simulink model "ECMO_Device_Project"  (R2020b)
settings: Solver=ode4  StartTime=0.0  StopTime=300  FixedStep=Tsamp  RelTol=1e-3
model workspace (MATLAB code in the model file):
  | %%%%%%%%%%%%%%%%%%%%%%%%%%%%%%%%%%%%%%%%%%%%%%%%%%%
  | %%%%%%%%%%%%% Term Project Parameters %%%%%%%%%%%%%
  | %%%%%%%%%%%%%%%%%%%%%%%%%%%%%%%%%%%%%%%%%%%%%%%%%%%
  | 
  | %% Physiological/Environmental Parameters
  | Tsamp = 1e-3;      % s
  | FIO2 = 50/100;  % (%) (Change this to 50% when ECMO is initiated)
  | FICO2 = 0.0/100;   % (%)
  | Patm = 760.0;      % mmHg
  | Pws = 47.0;        % mmHg
  | shunt = 36.5/100;  % (%)
  | 
  | %% Parameters of the Lung Mechanics
  | Clung = 0.062;     % l/cmH2O
  | Rtube = 3.76;      % cmH2O.s.l^-1
  | Rlung = 1.4013;    % cmH2O.s.l^-1
  | VL0 = 3.40;        % l
  | VReference = 0.2;  % l  (Change this to 0.2 l when ECMO is initiated)
  | 
  | %% Parameters of the Dead-Space
  | VD = 0.15;         % l
  | PdO2_IC = 60.0;    % mmHg
  | PdCO2_IC = 53.0;   % mmHg
  | 
  | %% Parameters of the Alveolar Gas Exchange
  | PAO2_IC = 57.0;    % mmHg
  | PACO2_IC = 55.0;   % mmHg
  | CaO2_IC = 0.184;   % ml/ml
  | CaCO2_IC = 0.565;  % ml/ml
  | Tau_TL = 10.0;     % s
  | kEff = 0.55;
  | 
  | %% Parameters of the Blood Dissociation Curves
  | CsatO2 = 0.2128;   % ml/ml
  | alpha1 = 0.03198;  % mmHg^-1
  | beta1 = 0.008275;  % mmHg^-1
  | K1 = 15.0;         % mmHg
  | h1 = 0.3836;
  | 
  | CsatCO2 = 1.9488;  % ml/ml
  | alpha2 = 0.05591;  % mmHg^-1
  | beta2 = 0.03255;   % mmHg^-1
  | K2 = 194.4;        % mmHg
  | h2 = 1.819;
  | 
  | %% Parameters of the Tissue Gas Exchange
  | VTO2 = 7700;       % ml
  | VTCO2 = 6000;      % ml
  | MRO2 = 3.80;       % ml/s
  | MRCO2 = 3.30;      % ml/s
  | CvO2_IC = 0.134;   % ml/ml
  | CvCO2_IC = 0.602;  % ml/ml
  | Tau_LT = 18.0;     % s
  | 
  | %% ECMO Pump Parameters
  | R = 10.0;     % ohm
  | L = 10.0;     % mH
  | kem = 0.192;  % V/(rd/s)
  | JL = 8e-4;    % kg.m^2
  | Ng = 0.5;
  | 
  | %% ECMO Oxygenator Parameters
  | VEO2 = 1.5;       % l
  | VECO2 = 1.5;      % l
  | PEO2_IC = 200.0;  % mmHg
  | PECO2_IC = 40.0;  % mmHg
  | 
  | FIEO2 = 100/100;   % (%)
  |  % (Change this to initiate ECMO)
libraries: fl_lib x19, nesl_utility x7, pid_lib x4
(part 1 of 2)
settings Model: OrderedModelArguments=off  Creator=kagan  LastModifiedBy=90535

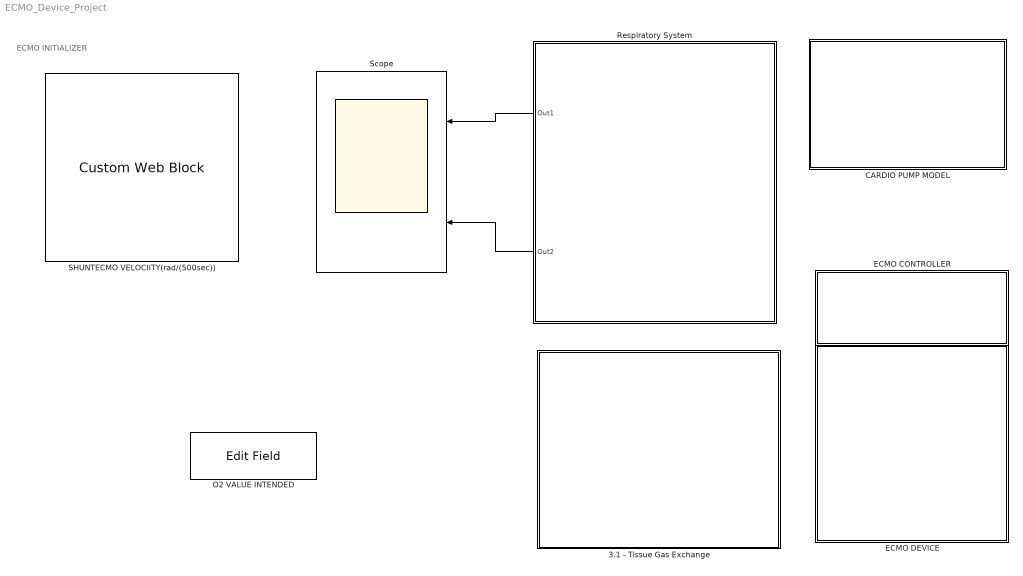
== system ECMO_Device_Project ==
  note: ECMO INITIALIZER
  3.1 - Tissue Gas Exchange : Subsystem
  CARDIO PUMP MODEL : Subsystem
  ECMO CONTROLLER : Subsystem
  ECMO DEVICE : Subsystem
  O2 VALUE INTENDED : EditField  LabelPosition=Hide  ShowInitialText=on  Alignment=Center
  Respiratory System : Subsystem
  SHUNTECMO VELOCIITY(rad/(500sec)) : CustomWebBlock  ShowInitialText=on  Configuration="{\"components\":[{\"name\":\"CircularScaleComponent\",\"settings\":{\"bounds\":{\"max\":1,\"min\":0,\"tickInterval\":\"auto\"},\"direction\":\"cw\",\"flipLimits\":0,\"innerRadius\":0.5069579852213397,\"internalTickHeightScaleFactor\":1,\"labelColor\":[250,245,200],\"labelFont\":{\"font\":\"Arial\",\"fontSize\":12},\"labelTransparency\":1,\"labelTrasparency\":1,\"minorTickHeightScaleFactor\":0.2,\"needleImage\":{\"size\":[200,50],\"src\":\"data:image\\/svg+xml;base64,PD94bWwgdmVyc2lvbj0iMS4wIiBlbmNvZGluZz0idXRmLTgiPz4KPCEtLSBHZW5lcmF0b3I6IEFkb2JlIElsbHVzdHJhdG9yIDE5LjIuMSwgU1ZHIEV4cG9ydCBQbHVnLUluIC4gU1ZHIFZlcnNpb246IDYuMDAgQnVpbGQgMCkgIC0tPgo8c3ZnIHZlcnNpb249IjEuMSIgeG1sbnM9Imh0dHA6Ly93d3cudzMub3JnLzIwMDAvc3ZnIiB4bWxuczp4bGluaz0iaHR0cDovL3d3dy53My5vcmcvMTk5OS94bGluayIgeD0iMHB4IiB5PSIwcHgiCgkgdmlld0JveD0iMCAwIDIwMCA1MCIgc3R5bGU9ImVuYWJsZS1iYWNrZ3JvdW5kOm5ldyAw ...(+9940 chars)\"},\"needleOffset\":[0.086575214380406,0],\"needleOrientation\":-45,\"needleRotation\":-180,\"needleSize\":{\"height\":0.09176649447596184,\"width\":0.3593006118373072},\"outerRadius\":0.6806022064516383,\"position\":[0.06486742424242424,0.05627705627705628,0.8917748917748918,0.8787878787878788],\"scaleAngle\":299.999999999988,\"scaleAngleOffset\":119.46147497096791,\"scaleColors\":[],\"scaleColorsSize\":0.2,\"scalePosition\":[0,0,1,1],\"showLabels\":1,\"showMinorTicks\":1,\"showSpanLine\":1,\"showTicks\":1,\"tickColor\":[250,245,200],\"tickTransparency\":1,\"valueBarColor\":[23,89,176],\"valueBarPosition\":[0,0,1,1],\"valueBarSize\":0.2,\"valueBarTransparency\":1}},{\"name\":\"BackgroundImageComponent\",\"settings\":{\"image\":{\"size\":[500,500],\"src\":\"data:image\\/svg+xml;base64,PD94bWwgdmVyc2lvbj0iMS4wIiBlbmNvZGluZz0iVVRGLTgiIHN0YW5kYWxvbmU9Im5vIj8+CjwhLS0gR2VuZXJhdG9yOiBBZG9iZSBJbGx1c3RyYXRvciAxOS4yLjEsIFNWRyBFeHBvcnQgUGx1Zy1JbiAuIFNWRyBWZXJzaW9uOiA2LjAwIEJ1aWxkIDApICAtLT4KCjxzdmcKICAgeG1sbnM6ZGM9Imh0dHA6Ly9wdXJsLm9yZy9kYy9lbGVtZW50cy8xLjEvIgogICB4bWxuczpjYz0iaHR0cDovL2NyZWF0aXZlY29tbW9ucy5vcmcvbnMjIgogICB4bWxuczpyZGY9Imh0dHA6Ly93d3cudzMub3JnLzE5OTkvMDIvMjItcmRmLXN5bnRh ...(+9660 chars)\",\"srcOrientation\":\"horizontal\"},\"position\":[0,0,1,1],\"scaleMode\":\"0\"}},{\"name\":\"ForegroundImageComponent\",\"settings\":{\"image\":{\"size\":[0,0],\"src\":\"default\",\"srcOrientation\":[]},\"isForeground\":1,\"position\":[0,0,1,1],\"scaleMode\":\"0\"}}],\"settings\":{\"BindingType\":\"signal\",\"aspectRatio\":1.0216110019646365,\"fixedAspectRatio\":\"on\",\"orientation\":\"horizontal\"},\"type\":\"CircularGauge\"}"
  Scope : Scope  NumInputPorts=2
  wires:
  Respiratory System/1(Out1) -> Scope/1
  Respiratory System/2(Out2) -> Scope/2

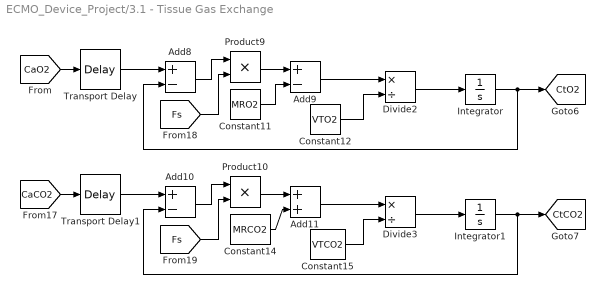
== system ECMO_Device_Project/3.1 - Tissue Gas Exchange ==
  Add10 : Sum  Inputs=+-
  Add11 : Sum
  Add8 : Sum  Inputs=+-
  Add9 : Sum  Inputs=+-
  Constant11 : Constant  Value=MRO2  SampleTime=Tsamp
  Constant12 : Constant  Value=VTO2  SampleTime=Tsamp
  Constant14 : Constant  Value=MRCO2  SampleTime=Tsamp
  Constant15 : Constant  Value=VTCO2  SampleTime=Tsamp
  Divide2 : Product  Inputs=*/
  Divide3 : Product  Inputs=*/
  Integrator : Integrator  InitialCondition=CvO2_IC
  Integrator1 : Integrator  InitialCondition=CvCO2_IC
  Product10 : Product
  Product9 : Product
  Transport Delay : TransportDelay  DelayTime=Tau_LT  InitialOutput=CaO2_IC
  Transport Delay1 : TransportDelay  DelayTime=Tau_LT  InitialOutput=CaCO2_IC
  tag scope: CtCO2=global, CtO2=global
  wires:
  [Fs] -> Product9/2
  Constant14/1 -> Add11/2
  [CaO2] -> Transport Delay/1
  Divide2/1 -> Integrator/1
  Integrator/1 -> Add8/2, [CtO2]
  Add8/1 -> Product9/1
  Add9/1 -> Divide2/1
  Divide3/1 -> Integrator1/1
  Constant12/1 -> Divide2/2
  Transport Delay/1 -> Add8/1
  Product9/1 -> Add9/1
  Constant11/1 -> Add9/2
  [CaCO2] -> Transport Delay1/1
  Integrator1/1 -> Add10/2, [CtCO2]
  Add11/1 -> Divide3/1
  Product10/1 -> Add11/1
  Transport Delay1/1 -> Add10/1
  Constant15/1 -> Divide3/2
  Add10/1 -> Product10/1
  [Fs] -> Product10/2

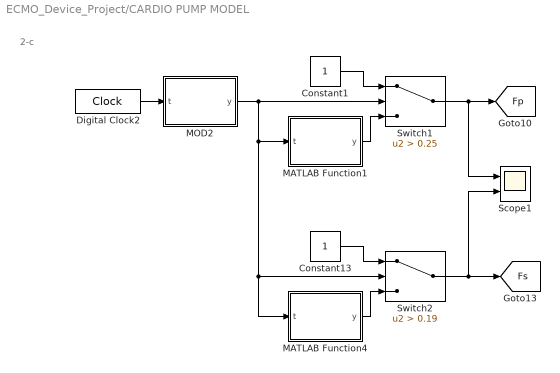
== system ECMO_Device_Project/CARDIO PUMP MODEL ==
  note: 2-c
  Constant1 : Constant
  Constant13 : Constant
  Digital Clock2 : DigitalClock  SampleTime=0.001
  MATLAB Function1 : MATLAB Function  TreatAsAtomicUnit=on
  MATLAB Function4 : MATLAB Function  TreatAsAtomicUnit=on
  MOD2 : MATLAB Function  TreatAsAtomicUnit=on
  Scope1 : Scope  NumInputPorts=2
  Switch1 : Switch  Criteria=u2 > Threshold  Threshold=0.25
  Switch2 : Switch  Criteria=u2 > Threshold  Threshold=0.19
  tag scope: Fp=global, Fs=global
  wires:
  Constant13/1 -> Switch2/1
  MOD2/1(y) -> MATLAB Function4/1(t), Switch2/2, MATLAB Function1/1(t), Switch1/2
  Switch1/1 -> [Fp], Scope1/1
  Switch2/1 -> Scope1/2, [Fs]
  Digital Clock2/1 -> MOD2/1(t)
  MATLAB Function4/1(y) -> Switch2/3
  Constant1/1 -> Switch1/1
  MATLAB Function1/1(y) -> Switch1/3

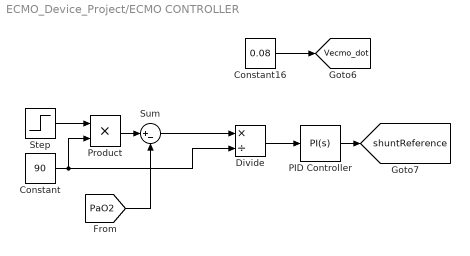
== system ECMO_Device_Project/ECMO CONTROLLER ==
  Constant : Constant  Value=90
  Constant16 : Constant  Value=0.08
  Divide : Product  Inputs=*/
  PID Controller : pid_lib/PID Controller  Controller=PI  Form=Parallel  TimeDomain=Continuous-time  UseExternalTs=off  SampleTime=-1  IntegratorMethod=Forward Euler  FilterMethod=Forward Euler  ControllerParametersSource=internal  P=10  I=4  D=600  UseFilter=on  N=100  TunerSelectOption=Transfer Function Based (PID Tuner App)  InitialConditionSource=internal  InitialConditionForIntegrator=0  InitialConditionForFilter=0  DifferentiatorICPrevScaledInput=0  ExternalReset=none  TrackingMode=off  Kt=1  LimitOutput=on  SatLimitsSource=internal  UpperSaturationLimit=1  LowerSaturationLimit=0  LinearizeAsGain=on  AntiWindupMode=none  Kb=1  POutMin=[]  POutMax=[]  IOutMin=[]  IOutMax=[]  DOutMin=[]  DOutMax=[]  NOutMin=[]  NOutMax=[]  SumOutMin=[]  SumOutMax=[]  SaturationOutMin=[]  SaturationOutMax=[]  PParamMin=[]  PParamMax=[]  IParamMin=[]  IParamMax=[]  DParamMin=[]  DParamMax=[]  NParamMin=[]  NParamMax=[]  KbParamMin=[]  KbParamMax=[]  KtParamMin=[]  KtParamMax=[]  KbOutMin=[]  KbOutMax=[]  KtOutMin=[]  KtOutMax=[]  IntegratorOutMin=[]  IntegratorOutMax=[]  FilterOutMin=[]  FilterOutMax=[]  SumI1OutMin=[]  SumI1OutMax=[]  SumI2OutMin=[]  SumI2OutMax=[]  SumI3OutMin=[]  SumI3OutMax=[]  SumI4OutMin=[]  SumI4OutMax=[]  SumDOutMin=[]  SumDOutMax=[]  DifferentiatorOutMin=[]  DifferentiatorOutMax=[]  FilterDiffOutCoefMin=[]  FilterDiffOutCoefMax=[]  ReciprocalOutMin=[]  ReciprocalOutMax=[]  SumDenOutMin=[]  SumDenOutMax=[]  SumNumOutMin=[]  SumNumOutMax=[]  DivideOutMin=[]  DivideOutMax=[]  UdiffTsProdOutMin=[]  UdiffTsProdOutMax=[]  NTsProdOutMin=[]  NTsProdOutMax=[]  UintegralTsProdOutMin=[]  UintegralTsProdOutMax=[]  UngainTsProdOutMin=[]  UngainTsProdOutMax=[]  IntegratorContinuousStateAttributes=''  IntegratorStateMustResolveToSignalObject=off  IntegratorRTWStateStorageClass=Auto  FilterContinuousStateAttributes=''  FilterStateMustResolveToSignalObject=off  FilterRTWStateStorageClass=Auto  ParallelPVariant=InternalParameters  IdealPVariant=Disabled  IVariant=InternalParameters  DVariant=Disabled  IntegratorVariant=Continuous  SatVariant=Enabled  AWVariant=Passthrough  PCopyVariant=Disabled  TRVariant=Disabled  FdbkBlocksVariant=Forward  IdealPFdbkVariant=Disabled  SatFdbkVariant=Disabled  DerivativeFilterVariant=Disabled  NVariant=Disabled  NCopyVariant=Disabled_SignalSpec  FilterICVariant=Disabled  IntegratorICVariant=InternalICs  ExternalResetVariant=Disabled  TRSumVariant=Passthrough  SumFdbkVariant=Disabled  SumVariant=Sum_PI  TsampFilterVariant=InternalTs  TsampNgainVariant=Passthrough  TsampIntegralVariant=Passthrough  ExternalSaturationOutDataTypeStr=Inherit: Same as second input
  Product : Product
  Step : Step  Time=0  SampleTime=0
  Sum : Sum  Inputs=|+-
  tag scope: Vecmo_dot=global, shuntReference=global
  wires:
  Product/1 -> Sum/1
  [PaO2] -> Sum/2
  PID Controller/1 -> [shuntReference]
  Constant16/1 -> [Vecmo_dot]
  Sum/1 -> Divide/1
  Divide/1 -> PID Controller/1
  Constant/1 -> Divide/2, Product/2
  Step/1 -> Product/1

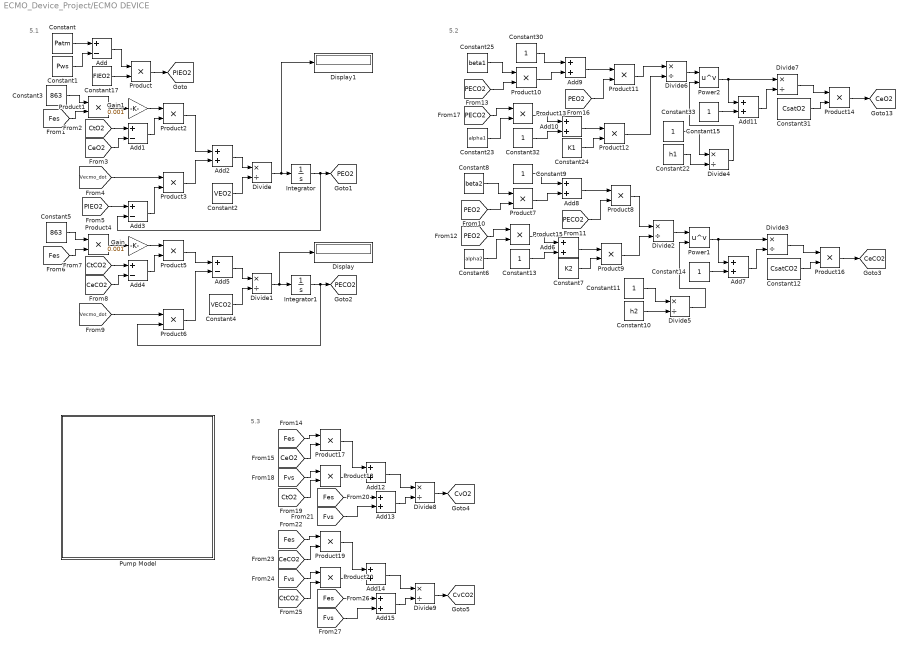
== system ECMO_Device_Project/ECMO DEVICE ==
  note: 5.3
  note: 5.1
  note: 5.2
  Add{,1,3..5} (5 alike) : Sum  Inputs=+-
  Add{2,6..15} (11 alike) : Sum
  Constant : Constant  Value=Patm
  Constant1 : Constant  Value=Pws
  Constant10 : Constant  Value=h2  SampleTime=Tsamp
  Constant{9,11,13..15,30,32..33} (8 alike) : Constant  SampleTime=Tsamp
  Constant12 : Constant  Value=CsatCO2  SampleTime=Tsamp
  Constant17 : Constant  Value=FIEO2
  Constant2 : Constant  Value=VEO2
  Constant22 : Constant  Value=h1  SampleTime=Tsamp
  Constant23 : Constant  Value=alpha1  SampleTime=Tsamp
  Constant24 : Constant  Value=K1  SampleTime=Tsamp
  Constant25 : Constant  Value=beta1  SampleTime=Tsamp
  Constant3 : Constant  Value=863
  Constant31 : Constant  Value=CsatO2  SampleTime=Tsamp
  Constant4 : Constant  Value=VECO2
  Constant5 : Constant  Value=863
  Constant6 : Constant  Value=alpha2  SampleTime=Tsamp
  Constant7 : Constant  Value=K2  SampleTime=Tsamp
  Constant8 : Constant  Value=beta2  SampleTime=Tsamp
  Display : Display
  Display1 : Display
  Divide{,1..9} (10 alike) : Product  Inputs=*/
  Gain : Gain  Gain=0.001
  Gain1 : Gain  Gain=0.001
  Integrator : Integrator  InitialCondition=PEO2_IC
  Integrator1 : Integrator  InitialCondition=PECO2_IC
  Power1 : Math  Operator=pow  SaturateOnIntegerOverflow=on
  Power2 : Math  Operator=pow  SaturateOnIntegerOverflow=on
  Product{,1..20} (21 alike) : Product
  "Pump Model " : Subsystem
  tag scope: CeCO2=global, CeO2=global, CvCO2=global, CvO2=global, PECO2=global, PEO2=global, PIEO2=global
  wires:
  [PECO2] -> Product8/2
  Constant2/1 -> Divide/2
  Product11/1 -> Divide6/1
  Divide4/1 -> Power2/2
  Constant15/1 -> Divide4/1
  Product7/1 -> Add8/2
  [Fes] -> Add13/1
  Add12/1 -> Divide8/1
  Gain/1 -> Product5/1
  Constant13/1 -> Add6/2
  Product20/1 -> Add14/2
  [Fvs] -> Add15/2
  [Fes] -> Product19/1
  Constant3/1 -> Product1/1
  [Fes] -> Product17/1
  [PECO2] -> Product10/2
  Power1/1 -> Add7/1, Divide3/1
  Add2/1 -> Divide/1
  Constant10/1 -> Divide5/2
  Add13/1 -> Divide8/2
  [CtO2] -> Product18/2
  Divide6/1 -> Power2/1
  Add3/1 -> Product3/2
  [PEO2] -> Product11/2
  Add10/1 -> Product12/1
  Divide1/1 -> Display/1, Integrator1/1
  [Fes] -> Product1/2
  Constant24/1 -> Product12/2
  Integrator1/1 -> Product6/2, [PECO2]
  Constant1/1 -> Add/2
  Constant6/1 -> Product15/2
  Integrator/1 -> Add3/2, [PEO2]
  Add11/1 -> Divide7/2
  Product8/1 -> Divide2/1
  Product17/1 -> Add12/1
  [Vecmo_dot] -> Product3/1
  [CtCO2] -> Add4/1
  Constant7/1 -> Product9/2
  Product18/1 -> Add12/2
  Product10/1 -> Add9/2
  Product14/1 -> [CeO2]
  Add4/1 -> Product5/2
  [PIEO2] -> Add3/1
  Product6/1 -> Add5/2
  Constant14/1 -> Add7/2
  Divide5/1 -> Power1/2
  Gain1/1 -> Product2/1
  Add9/1 -> Product11/1
  Product5/1 -> Add5/1
  Constant33/1 -> Add11/2
  Add15/1 -> Divide9/2
  Add8/1 -> Product8/1
  Constant11/1 -> Divide5/1
  [PEO2] -> Product15/1
  Constant5/1 -> Product4/1
  Constant17/1 -> Product/2
  Constant31/1 -> Product14/2
  Divide3/1 -> Product16/1
  Divide/1 -> Display1/1, Integrator/1
  Add1/1 -> Product2/2
  Add7/1 -> Divide3/2
  Add/1 -> Product/1
  Constant/1 -> Add/1
  Power2/1 -> Add11/1, Divide7/1
  Add5/1 -> Divide1/1
  Constant12/1 -> Product16/2
  Product9/1 -> Divide2/2
  Product16/1 -> [CeCO2]
  Constant32/1 -> Add10/2
  Product12/1 -> Divide6/2
  Product3/1 -> Add2/2
  Divide2/1 -> Power1/1
  [Fvs] -> Product18/1
  [CeCO2] -> Product19/2
  [Fes] -> Product4/2
  Add14/1 -> Divide9/1
  Divide8/1 -> [CvO2]
  Constant9/1 -> Add8/1
  [CtO2] -> Add1/1
  [Fvs] -> Add13/2
  Divide7/1 -> Product14/1
  Constant4/1 -> Divide1/2
  Divide9/1 -> [CvCO2]
  Constant8/1 -> Product7/1
  Add6/1 -> Product9/1
  Product1/1 -> Gain1/1
  Constant30/1 -> Add9/1
  Product2/1 -> Add2/1
  Product15/1 -> Add6/1
  Product/1 -> [PIEO2]
  Constant25/1 -> Product10/1
  [PECO2] -> Product13/1
  Constant23/1 -> Product13/2
  [CeO2] -> Product17/2
  Product4/1 -> Gain/1
  Product13/1 -> Add10/1
  [Fvs] -> Product20/1
  Constant22/1 -> Divide4/2
  [CeO2] -> Add1/2
  [PEO2] -> Product7/2
  [Vecmo_dot] -> Product6/1
  [CeCO2] -> Add4/2
  [CtCO2] -> Product20/2
  [Fes] -> Add15/1
  Product19/1 -> Add14/1

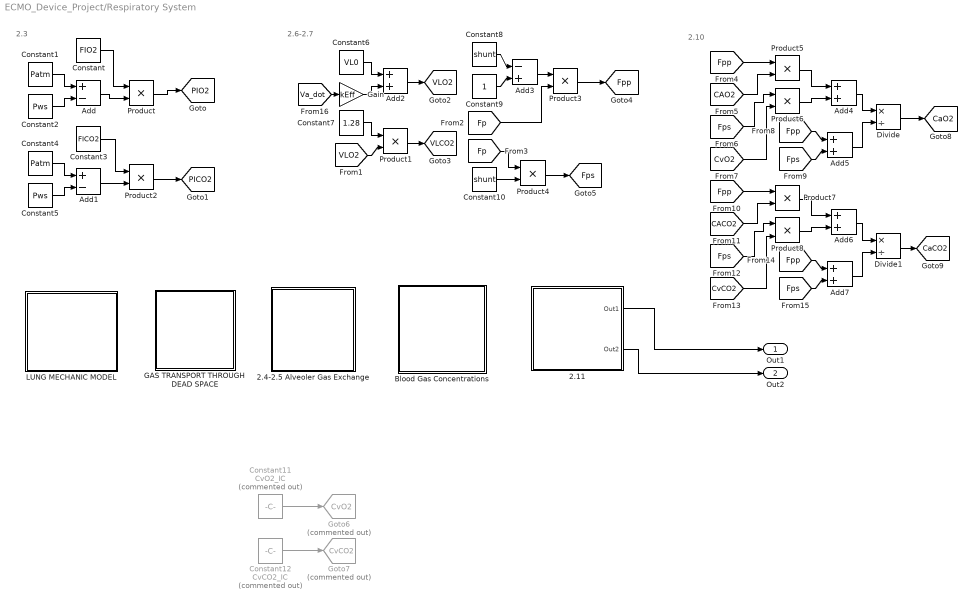
== system ECMO_Device_Project/Respiratory System ==
  note: 2.10
  note: 2.6-2.7
  note: 2.3
  "2.11 " : Subsystem
  2.4-2.5 Alveoler Gas Exchange : Subsystem
  Add : Sum  Inputs=+-
  Add1 : Sum  Inputs=+-
  Add{2,4..7} (5 alike) : Sum
  Add3 : Sum  Inputs=-+
  "Blood Gas Concentrations " : Subsystem
  Constant : Constant  Value=FIO2  SampleTime=Tsamp
  Constant1 : Constant  Value=Patm  SampleTime=Tsamp
  Constant10 : Constant  Value=shunt  SampleTime=Tsamp
  Constant11 : Constant  Commented=on  Value=CvO2_IC  SampleTime=Tsamp
  Constant12 : Constant  Commented=on  Value=CvCO2_IC  SampleTime=Tsamp
  Constant2 : Constant  Value=Pws  SampleTime=Tsamp
  Constant3 : Constant  Value=FICO2  SampleTime=Tsamp
  Constant4 : Constant  Value=Patm  SampleTime=Tsamp
  Constant5 : Constant  Value=Pws  SampleTime=Tsamp
  Constant6 : Constant  Value=VL0  SampleTime=Tsamp
  Constant7 : Constant  Value=1.28  SampleTime=Tsamp
  Constant8 : Constant  Value=shunt  SampleTime=Tsamp
  Constant9 : Constant  SampleTime=Tsamp
  Divide : Product  Inputs=*/
  Divide1 : Product  Inputs=*/
  GAS TRANSPORT THROUGH DEAD SPACE : Subsystem
  Gain : Gain  Gain=kEff
  Goto6 : Goto  Commented=on  GotoTag=CvO2  TagVisibility=global
  Goto7 : Goto  Commented=on  GotoTag=CvCO2  TagVisibility=global
  LUNG MECHANIC MODEL : Subsystem
  Product{,1..8} (9 alike) : Product
  Out1 : Outport
  Out2 : Outport  Port=2
  tag scope: CaCO2=global, CaO2=global, Fpp=global, Fps=global, PICO2=global, PIO2=global, VLCO2=global, VLO2=global
  wires:
  Constant9/1 -> Add3/2
  Add5/1 -> Divide/2
  Constant2/1 -> Add/2
  Constant10/1 -> Product4/2
  Constant8/1 -> Add3/1
  Add4/1 -> Divide/1
  [Fp] -> Product3/2
  Add2/1 -> [VLO2]
  [CvO2] -> Product6/2
  Constant5/1 -> Add1/2
  Constant7/1 -> Product1/1
  [VLO2] -> Product1/2
  Constant3/1 -> Product2/1
  [Fp] -> Product4/1
  Add3/1 -> Product3/1
  Constant1/1 -> Add/1
  Product5/1 -> Add4/1
  Product8/1 -> Add6/2
  Constant4/1 -> Add1/1
  Product3/1 -> [Fpp]
  Gain/1 -> Add2/2
  [Fps] -> Add7/2
  Product1/1 -> [VLCO2]
  [Fpp] -> Add7/1
  Product2/1 -> [PICO2]
  Add/1 -> Product/2
  Add1/1 -> Product2/2
  Constant6/1 -> Add2/1
  Add6/1 -> Divide1/1
  [CvCO2] -> Product8/2
  [CACO2] -> Product7/2
  Product6/1 -> Add4/2
  [CAO2] -> Product5/2
  Product4/1 -> [Fps]
  [Fpp] -> Add5/1
  Constant/1 -> Product/1
  Product7/1 -> Add6/1
  Divide1/1 -> [CaCO2]
  Product/1 -> [PIO2]
  [Va_dot] -> Gain/1
  [Fps] -> Product8/1
  [Fpp] -> Product5/1
  [Fps] -> Add5/2
  Add7/1 -> Divide1/2
  [Fps] -> Product6/1
  [Fpp] -> Product7/1
  Divide/1 -> [CaO2]
  Constant11/1 -> Goto6/1
  Constant12/1 -> Goto7/1
  "2.11 "/1(Out1) -> Out1/1
  "2.11 "/2(Out2) -> Out2/1

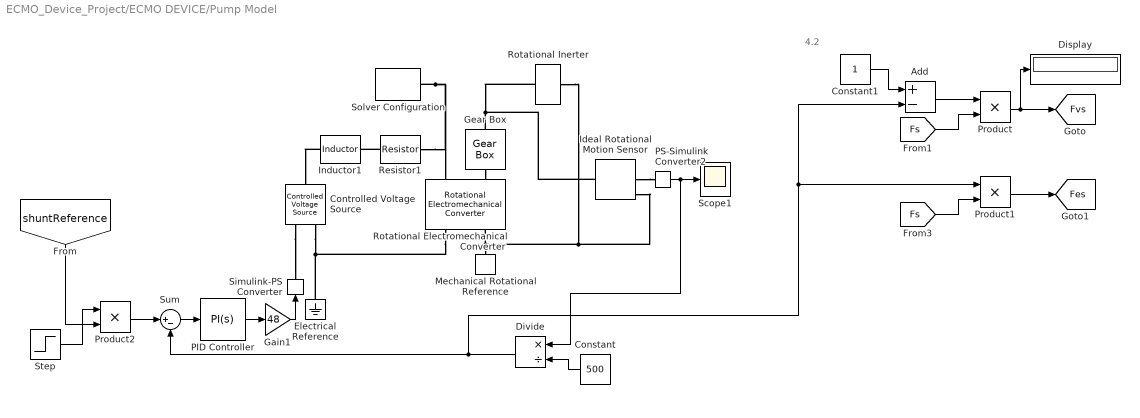
== system ECMO_Device_Project/ECMO DEVICE/Pump Model  ==
  note: 4.2
  Add : Sum  Inputs=+-
  Constant : Constant  Value=500
  Constant1 : Constant
  Controlled Voltage Source : fl_lib/Electrical/Electrical Sources/Controlled Voltage Source
  Display : Display
  Divide : Product  Inputs=*/
  Electrical Reference : fl_lib/Electrical/Electrical Elements/Electrical Reference
  Gain1 : Gain  Gain=48
  Gear Box : fl_lib/Mechanical/Mechanisms/Gear Box  ratio=Ng  t_in_specify=off  t_in_priority=None  t_in=0 N*m  t_in_nominal_specify=off  t_in_nominal_unit=N*m  t_in_nominal_value=1  t_out_specify=off  t_out_priority=None  t_out=0 N*m  t_out_nominal_specify=off  t_out_nominal_unit=N*m  t_out_nominal_value=1
  Ideal Rotational Motion Sensor : fl_lib/Mechanical/Mechanical Sensors/Ideal Rotational Motion Sensor  wrap_angle=simscape.enum.onoff.off  offset=0 rad
  Inductor1 : fl_lib/Electrical/Electrical Elements/Inductor  l=L mH  r=0 Ohm  g=1e-9 1/Ohm  i_specify=off  i_priority=None  i=0 A  i_nominal_specify=off  i_nominal_unit=A  i_nominal_value=1  v_specify=off  v_priority=None  v=0 V  v_nominal_specify=off  v_nominal_unit=V  v_nominal_value=1  i_L_specify=off  i_L_priority=High  i_L=0 A  i_L_nominal_specify=off  i_L_nominal_unit=A  i_L_nominal_value=1
  Mechanical Rotational Reference : fl_lib/Mechanical/Rotational Elements/Mechanical Rotational Reference
  PID Controller : pid_lib/PID Controller  Controller=PI  Form=Parallel  TimeDomain=Continuous-time  UseExternalTs=off  SampleTime=-1  IntegratorMethod=Forward Euler  FilterMethod=Forward Euler  ControllerParametersSource=internal  P=300  I=48.35  D=0  UseFilter=on  N=100  TunerSelectOption=Transfer Function Based (PID Tuner App)  InitialConditionSource=internal  InitialConditionForIntegrator=0  InitialConditionForFilter=0  DifferentiatorICPrevScaledInput=0  ExternalReset=none  TrackingMode=off  Kt=1  LimitOutput=on  SatLimitsSource=internal  UpperSaturationLimit=1  LowerSaturationLimit=0  LinearizeAsGain=on  AntiWindupMode=none  Kb=1  POutMin=[]  POutMax=[]  IOutMin=[]  IOutMax=[]  DOutMin=[]  DOutMax=[]  NOutMin=[]  NOutMax=[]  SumOutMin=[]  SumOutMax=[]  SaturationOutMin=[]  SaturationOutMax=[]  PParamMin=[]  PParamMax=[]  IParamMin=[]  IParamMax=[]  DParamMin=[]  DParamMax=[]  NParamMin=[]  NParamMax=[]  KbParamMin=[]  KbParamMax=[]  KtParamMin=[]  KtParamMax=[]  KbOutMin=[]  KbOutMax=[]  KtOutMin=[]  KtOutMax=[]  IntegratorOutMin=[]  IntegratorOutMax=[]  FilterOutMin=[]  FilterOutMax=[]  SumI1OutMin=[]  SumI1OutMax=[]  SumI2OutMin=[]  SumI2OutMax=[]  SumI3OutMin=[]  SumI3OutMax=[]  SumI4OutMin=[]  SumI4OutMax=[]  SumDOutMin=[]  SumDOutMax=[]  DifferentiatorOutMin=[]  DifferentiatorOutMax=[]  FilterDiffOutCoefMin=[]  FilterDiffOutCoefMax=[]  ReciprocalOutMin=[]  ReciprocalOutMax=[]  SumDenOutMin=[]  SumDenOutMax=[]  SumNumOutMin=[]  SumNumOutMax=[]  DivideOutMin=[]  DivideOutMax=[]  UdiffTsProdOutMin=[]  UdiffTsProdOutMax=[]  NTsProdOutMin=[]  NTsProdOutMax=[]  UintegralTsProdOutMin=[]  UintegralTsProdOutMax=[]  UngainTsProdOutMin=[]  UngainTsProdOutMax=[]  IntegratorContinuousStateAttributes=''  IntegratorStateMustResolveToSignalObject=off  IntegratorRTWStateStorageClass=Auto  FilterContinuousStateAttributes=''  FilterStateMustResolveToSignalObject=off  FilterRTWStateStorageClass=Auto  ParallelPVariant=InternalParameters  IdealPVariant=Disabled  IVariant=InternalParameters  DVariant=Disabled  IntegratorVariant=Continuous  SatVariant=Enabled  AWVariant=Passthrough  PCopyVariant=Disabled  TRVariant=Disabled  FdbkBlocksVariant=Forward  IdealPFdbkVariant=Disabled  SatFdbkVariant=Disabled  DerivativeFilterVariant=Disabled  NVariant=Disabled  NCopyVariant=Disabled_SignalSpec  FilterICVariant=Disabled  IntegratorICVariant=InternalICs  ExternalResetVariant=Disabled  TRSumVariant=Passthrough  SumFdbkVariant=Disabled  SumVariant=Sum_PI  TsampFilterVariant=InternalTs  TsampNgainVariant=Passthrough  TsampIntegralVariant=Passthrough  ExternalSaturationOutDataTypeStr=Inherit: Same as second input
  PS-Simulink Converter2 : nesl_utility/PS-Simulink Converter  PhysicalDomain=network_engine_domain  SubClassName=ps_output  LeftPortType=input  RightPortType=output  PseudoPeriodic=off  Frequencies=[]  Unit=inherit  AffineConversion=off
  Product : Product
  Product1 : Product
  Product2 : Product
  Resistor1 : fl_lib/Electrical/Electrical Elements/Resistor  R=R Ohm  i_specify=off  i_priority=None  i=0 A  i_nominal_specify=off  i_nominal_unit=A  i_nominal_value=1  v_specify=off  v_priority=None  v=0 V  v_nominal_specify=off  v_nominal_unit=V  v_nominal_value=1
  Rotational Electromechanical Converter : fl_lib/Electrical/Electrical Elements/Rotational Electromechanical Converter  K=kem V/(rad/s)  i_specify=off  i_priority=None  i=0 A  i_nominal_specify=off  i_nominal_unit=A  i_nominal_value=1  v_specify=off  v_priority=None  v=0 V  v_nominal_specify=off  v_nominal_unit=V  v_nominal_value=1  t_specify=off  t_priority=None  t=0 N*m  t_nominal_specify=off  t_nominal_unit=N*m  t_nominal_value=1  w_specify=off  w_priority=None  w=0 rad/s  w_nominal_specify=off  w_nominal_unit=rad/s  w_nominal_value=1
  Rotational Inerter : fl_lib/Mechanical/Rotational Elements/Rotational Inerter  B=JL kg*m^2  w_specify=off  w_priority=High  w=0 rad/s  w_nominal_specify=off  w_nominal_unit=rad/s  w_nominal_value=1  t_specify=off  t_priority=None  t=0 N*m  t_nominal_specify=off  t_nominal_unit=N*m  t_nominal_value=1
      settings: SourceProductBaseCode=SS  InternalSimscapePortConfiguration="{\"Bottom\":[],\"Left\":[{\"id\":\"R\",\"label\":\"R\",\"type\":\"foundation.mechanical.rotational.rotational\"}],\"Right\":[{\"id\":\"C\",\"label\":\"C\",\"type\":\"foundation.mechanical.rotational.rotational\"}],\"Top\":[]}"
  Scope1 : Scope
  Simulink-PS Converter : nesl_utility/Simulink-PS Converter  PhysicalDomain=network_engine_domain  SubClassName=ps_input  LeftPortType=input  RightPortType=output  PseudoPeriodic=off  Frequencies=[]  NoiseDistribution=none  NoiseParameters=[]  Unit=1  AffineConversion=off  FilteringAndDerivatives=provide  SimscapeFilterOrder=1  InputFilterTimeConstant=0.001  UdotUserProvided=0
  Solver Configuration : nesl_utility/Solver Configuration  PhysicalDomain=network_engine_domain  SubClassName=solver  LeftPortType=input  RightPortType=generic  Tones=[]  Harmonics=[]  SimulateNoise=off  Profile=off  UseLocalSampling=off  EnableSwitchedLinearOptims=on  FrequencyDomain=off  UseCCode=off  RelTol=0.001  AbsTol=1e-06  MinStep=1e-09  ToWorkspace=off  RevertToSquareIcSolve=off  NumHomotopyIterations=100  PhasorMode=off  PhasorModeNumHarmonics=1  DoDC=off  ResidualTolerance=1e-09  UseLocalSolver=off  LocalSolverChoice=NE_BACKWARD_EULER_ADVANCER  LocalSolverSampleTime=0.001  DoFixedCost=off  MaxNonlinIter=3  MaxModeIter=2  ComputeImpulses=off  ImpulseIterations=2  LinearAlgebra=auto  EquationFormulation=NE_TIME_EF  DelaysMemoryBudget=1024  AutomaticFiltering=on  FilteringTimeConstant=0.001  PartitionStorageMethod=AS_NEEDED  PartitionMemoryBudget=1024  PartitionMethod=ROBUST
  Step : Step  Time=0  SampleTime=0
  Sum : Sum  Inputs=|+-
  tag scope: Fes=global, Fvs=global
  wires:
  Sum/1 -> PID Controller/1
  Gain1/1 -> Simulink-PS Converter/1
  Constant/1 -> Divide/2
  PS-Simulink Converter2/1 -> Scope1/1, Divide/1
  Product2/1 -> Sum/1
  Step/1 -> Product2/1
  Divide/1 -> Product1/1, Add/2, Sum/2
  Constant1/1 -> Add/1
  Add/1 -> Product/1
  [Fs] -> Product/2
  Product/1 -> Display/1, [Fvs]
  PID Controller/1 -> Gain1/1
  [Fs] -> Product1/2
  Product1/1 -> [Fes]
  [shuntReference] -> Product2/2
  connections:
  Ideal Rotational Motion Sensor/RConn1 -- Mechanical Rotational Reference/LConn1 -- Rotational Electromechanical Converter/RConn2 -- Rotational Inerter/RConn1
  Controlled Voltage Source/RConn2 -- Rotational Electromechanical Converter/RConn1 -- Electrical Reference/LConn1
  Gear Box/LConn1 -- Rotational Electromechanical Converter/LConn2
  Gear Box/RConn1 -- Rotational Inerter/LConn1 -- Ideal Rotational Motion Sensor/LConn1
  Solver Configuration/RConn1 -- Resistor1/RConn1 -- Rotational Electromechanical Converter/LConn1
  Ideal Rotational Motion Sensor/RConn2 -- PS-Simulink Converter2/LConn1
  Inductor1/LConn1 -- Controlled Voltage Source/LConn1
  Controlled Voltage Source/RConn1 -- Simulink-PS Converter/RConn1
  Resistor1/LConn1 -- Inductor1/RConn1

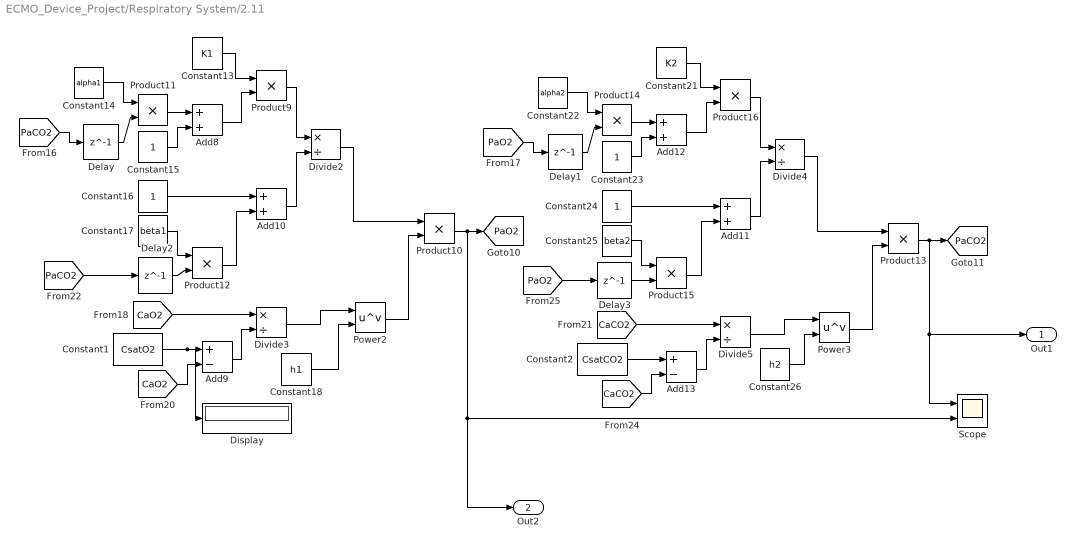
== system ECMO_Device_Project/Respiratory System/2.11  ==
  Add{8,10..12} (4 alike) : Sum
  Add13 : Sum  Inputs=+-
  Add9 : Sum  Inputs=+-
  Constant1 : Constant  Value=CsatO2  SampleTime=Tsamp
  Constant13 : Constant  Value=K1  SampleTime=Tsamp
  Constant14 : Constant  Value=alpha1  SampleTime=Tsamp
  Constant{15..16,23..24} (4 alike) : Constant  SampleTime=Tsamp
  Constant17 : Constant  Value=beta1  SampleTime=Tsamp
  Constant18 : Constant  Value=h1  SampleTime=Tsamp
  Constant2 : Constant  Value=CsatCO2  SampleTime=Tsamp
  Constant21 : Constant  Value=K2  SampleTime=Tsamp
  Constant22 : Constant  Value=alpha2  SampleTime=Tsamp
  Constant25 : Constant  Value=beta2  SampleTime=Tsamp
  Constant26 : Constant  Value=h2  SampleTime=Tsamp
  Delay : Delay  DelayLength=1  SampleTime=Tsamp
  Delay1 : Delay  DelayLength=1  InitialCondition=0  SampleTime=Tsamp
  Delay2 : Delay  DelayLength=1  InitialCondition=0  SampleTime=Tsamp
  Delay3 : Delay  DelayLength=1  InitialCondition=0  SampleTime=Tsamp
  Display : Display
  Divide{2..5} (4 alike) : Product  Inputs=*/
  Power2 : Math  Operator=pow  SaturateOnIntegerOverflow=on
  Power3 : Math  Operator=pow  SaturateOnIntegerOverflow=on
  Product{9..16} (8 alike) : Product
  Scope : Scope  NumInputPorts=2
  Out1 : Outport
  Out2 : Outport  Port=2
  tag scope: PaCO2=global, PaO2=global
  wires:
  Constant2/1 -> Add13/1
  Constant22/1 -> Product14/1
  [CaO2] -> Divide3/1
  Divide4/1 -> Product13/1
  Constant21/1 -> Product16/1
  Constant15/1 -> Add8/2
  Add12/1 -> Product16/2
  Add10/1 -> Divide2/2
  Product13/1 -> Out1/1, Scope/1, [PaCO2]
  Constant1/1 -> Display/1, Add9/1
  Add13/1 -> Divide5/2
  Product15/1 -> Add11/2
  Constant25/1 -> Product15/1
  [PaCO2] -> Delay/1
  Constant24/1 -> Add11/1
  Delay/1 -> Product11/2
  Delay1/1 -> Product14/2
  Product11/1 -> Add8/1
  [PaO2] -> Delay1/1
  Product10/1 -> Out2/1, Scope/2, [PaO2]
  [CaCO2] -> Add13/2
  Product12/1 -> Add10/2
  Product16/1 -> Divide4/1
  Constant14/1 -> Product11/1
  Power3/1 -> Product13/2
  Constant23/1 -> Add12/2
  [CaCO2] -> Divide5/1
  Add11/1 -> Divide4/2
  Product14/1 -> Add12/1
  Constant17/1 -> Product12/1
  Constant16/1 -> Add10/1
  Constant13/1 -> Product9/1
  Product9/1 -> Divide2/1
  Power2/1 -> Product10/2
  Add8/1 -> Product9/2
  [CaO2] -> Add9/2
  Divide2/1 -> Product10/1
  Add9/1 -> Divide3/2
  [PaCO2] -> Delay2/1
  Delay2/1 -> Product12/2
  Divide3/1 -> Power2/1
  Constant18/1 -> Power2/2
  Divide5/1 -> Power3/1
  Constant26/1 -> Power3/2
  [PaO2] -> Delay3/1
  Delay3/1 -> Product15/2

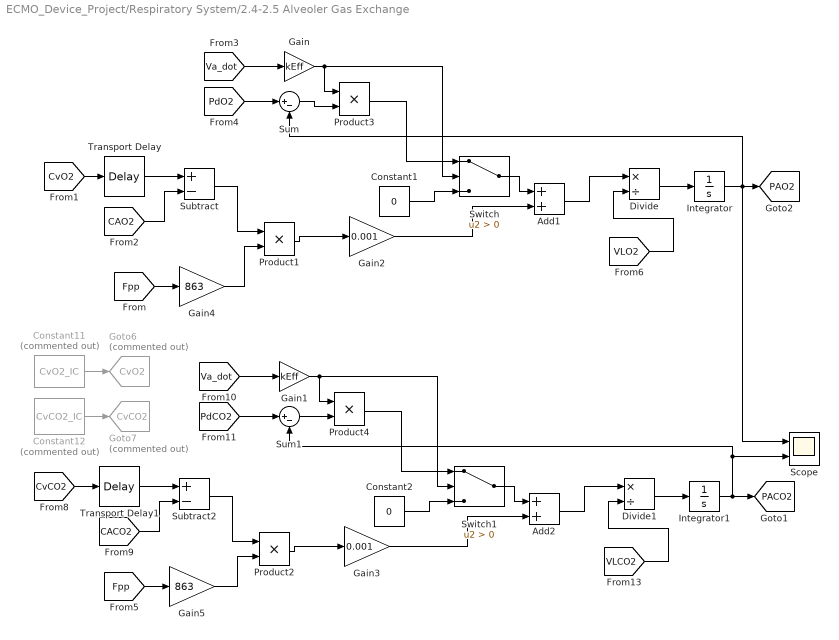
== system ECMO_Device_Project/Respiratory System/2.4-2.5 Alveoler Gas Exchange ==
  Add1 : Sum
  Add2 : Sum
  Constant1 : Constant  Value=0  SampleTime=Tsamp
  Constant11 : Constant  Commented=on  Value=CvO2_IC  SampleTime=Tsamp
  Constant12 : Constant  Commented=on  Value=CvCO2_IC  SampleTime=Tsamp
  Constant2 : Constant  Value=0  SampleTime=Tsamp
  Divide : Product  Inputs=*/
  Divide1 : Product  Inputs=*/
  Gain : Gain  Gain=kEff
  Gain1 : Gain  Gain=kEff
  Gain2 : Gain  Gain=0.001
  Gain3 : Gain  Gain=0.001
  Gain4 : Gain  Gain=863
  Gain5 : Gain  Gain=863
  Goto6 : Goto  Commented=on  GotoTag=CvO2  TagVisibility=global
  Goto7 : Goto  Commented=on  GotoTag=CvCO2  TagVisibility=global
  Integrator : Integrator  InitialCondition=PAO2_IC
  Integrator1 : Integrator  InitialCondition=PACO2_IC
  Product{1..4} (4 alike) : Product
  Scope : Scope  NumInputPorts=2
  Subtract : Sum  Inputs=+-
  Subtract2 : Sum  Inputs=+-
  Sum : Sum  Inputs=|+-
  Sum1 : Sum  Inputs=|+-
  Switch : Switch  Criteria=u2 > Threshold
  Switch1 : Switch  Criteria=u2 > Threshold
  Transport Delay : TransportDelay  DelayTime=Tau_TL  InitialOutput=CvO2_IC  BufferSize=10240  FixedBuffer=on
  Transport Delay1 : TransportDelay  DelayTime=Tau_TL  InitialOutput=CvCO2_IC  BufferSize=10240  FixedBuffer=on
  tag scope: PACO2=global, PAO2=global
  wires:
  Product3/1 -> Switch/1
  Subtract/1 -> Product1/1
  [CAO2] -> Subtract/2
  [Va_dot] -> Gain/1
  Gain/1 -> Product3/1, Switch/2
  Transport Delay/1 -> Subtract/1
  [CvO2] -> Transport Delay/1
  Divide/1 -> Integrator/1
  [PdO2] -> Sum/1
  Integrator/1 -> Sum/2, Scope/1, [PAO2]
  Sum/1 -> Product3/2
  [VLO2] -> Divide/2
  Product1/1 -> Gain2/1
  Constant1/1 -> Switch/3
  Switch/1 -> Add1/1
  Gain2/1 -> Add1/2
  Add1/1 -> Divide/1
  [PdCO2] -> Sum1/1
  [CvCO2] -> Transport Delay1/1
  Subtract2/1 -> Product2/1
  [CACO2] -> Subtract2/2
  Divide1/1 -> Integrator1/1
  Switch1/1 -> Add2/1
  Integrator1/1 -> Sum1/2, Scope/2, [PACO2]
  Transport Delay1/1 -> Subtract2/1
  Sum1/1 -> Product4/2
  Product4/1 -> Switch1/1
  Constant2/1 -> Switch1/3
  [VLCO2] -> Divide1/2
  Product2/1 -> Gain3/1
  Add2/1 -> Divide1/1
  [Va_dot] -> Gain1/1
  Gain3/1 -> Add2/2
  Gain1/1 -> Product4/1, Switch1/2
  [Fpp] -> Gain4/1
  Gain4/1 -> Product1/2
  Gain5/1 -> Product2/2
  [Fpp] -> Gain5/1
  Constant12/1 -> Goto7/1
  Constant11/1 -> Goto6/1
